simulink model "ex_3_water"  (R2018a)
settings: Solver=VariableStepAuto  StartTime=0.0  StopTime=100  RelTol=1e-3
libraries: simulink x1
settings Model: Creator=k2202936  LastModifiedBy=k2202936

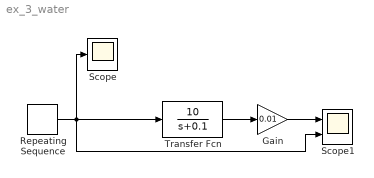
== system ex_3_water ==
  Gain : Gain  Gain=0.01
  Repeating Sequence : simulink/Sources/Repeating Sequence  rep_seq_t=[0 10 50 60 100]  rep_seq_y=[0 10 10 0 0]
  Scope : Scope
  Scope1 : Scope  NumInputPorts=2
  Transfer Fcn : TransferFcn  Numerator=[10]  Denominator=[1 0.1]
  wires:
  Repeating Sequence/1 -> Scope1/2, Scope/1, Transfer Fcn/1
  Transfer Fcn/1 -> Gain/1
  Gain/1 -> Scope1/1
